simulink subsystem "ROS2"  (R2024b)
settings: Solver=VariableStepAuto  StartTime=0.0  StopTime=10.0  RelTol=1e-3
settings Model: Creator=macheson  LastModifiedBy=macheson

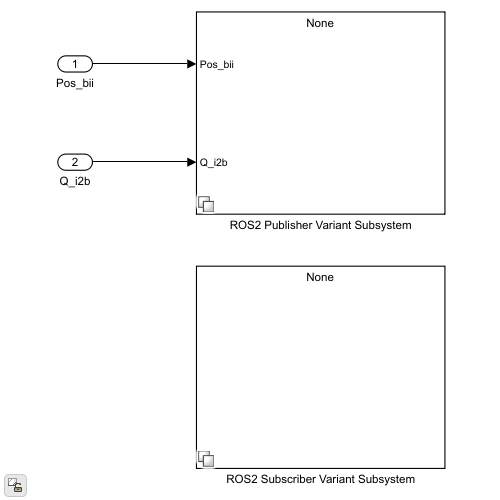
[thumbnail: Simulink's stored preview of the top-level diagram]
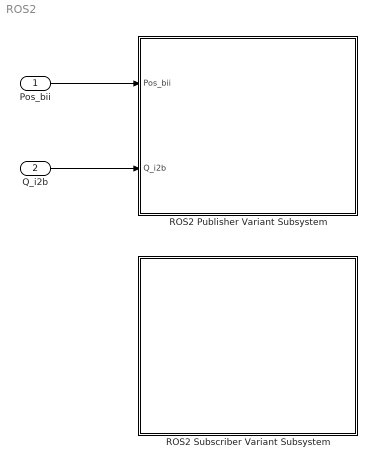
== system ROS2 ==
  Pos_bii : Inport
  Q_i2b : Inport  Port=2
  ROS2 Publisher Variant Subsystem : Subsystem  Variant=on
  ROS2 Subscriber Variant Subsystem : Subsystem  Variant=on
  wires:
  Q_i2b/1 -> ROS2 Publisher Variant Subsystem/2(Q_i2b)
  Pos_bii/1 -> ROS2 Publisher Variant Subsystem/1(Pos_bii)

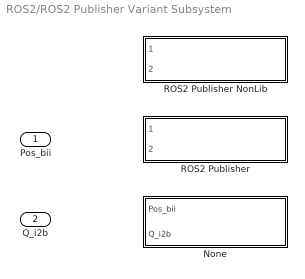
== system ROS2/ROS2 Publisher Variant Subsystem ==
  Pos_bii : Inport
  Q_i2b : Inport  Port=2
  None : Subsystem  VariantControl=PUB_TYPE_NONE
  ROS2 Publisher : Subsystem  VariantControl=PUB_TYPE_ROS2  ReferencedSubsystem=ROS2_MatPub
  ROS2 Publisher NonLib : Subsystem  VariantControl=PUB_TYPE_ROS2_NONLIB  ReferencedSubsystem=ROS2_MatPub_NonLib

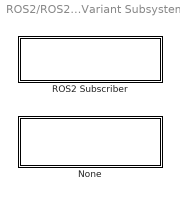
== system ROS2/ROS2 Subscriber Variant Subsystem ==
  None : Subsystem  VariantControl=SUB_TYPE_NONE
  ROS2 Subscriber : Subsystem  VariantControl=SUB_TYPE_PHASE  ReferencedSubsystem=ROS2_MatSub

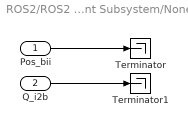
== system ROS2/ROS2 Publisher Variant Subsystem/None ==
  Pos_bii : Inport
  Q_i2b : Inport  Port=2
  Terminator : Terminator
  Terminator1 : Terminator
  wires:
  Pos_bii/1 -> Terminator/1
  Q_i2b/1 -> Terminator1/1

== system ROS2/ROS2 Subscriber Variant Subsystem/None ==
